simulink model "Lab6_dyskretny"  (R2017a)
settings: Solver=VariableStepAuto  StartTime=0.0  StopTime=10.0  FixedStep=0.01  RelTol=1e-3
values from neighbouring files (symbols this model uses):
  h = bodeplot(K)    [Lab1.m]    (also in Lab5.m = nyquistplot(K0); Lab6.m = h1)
libraries: cstblocks x2
settings Model: Creator=ishiguro  LastModifiedBy=ishiguro
settings DataIOCC: TimeSaveName=tout_dysk

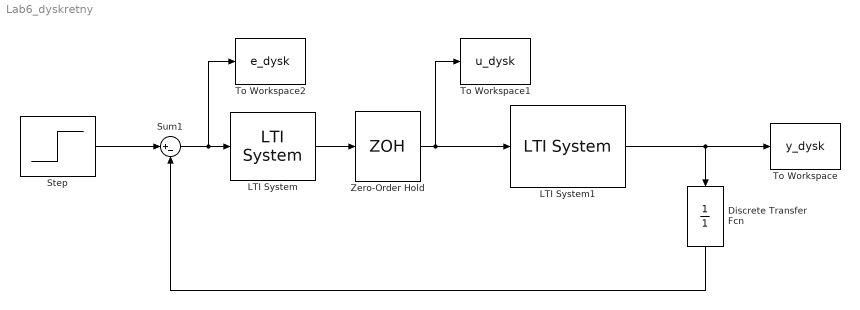
== system Lab6_dyskretny ==
  Discrete Transfer Fcn : DiscreteTransferFcn  Denominator=[1]  SampleTime=h
  LTI System : cstblocks/LTI System  sys=Kr  IC=[]
  LTI System1 : cstblocks/LTI System  sys=K  IC=[]
  Step : Step  Time=0  SampleTime=0
  Sum1 : Sum  Inputs=|+-
  To Workspace : ToWorkspace  VariableName=y_dysk  SampleTime=-1
  To Workspace1 : ToWorkspace  VariableName=u_dysk  SampleTime=-1
  To Workspace2 : ToWorkspace  VariableName=e_dysk  SampleTime=-1
  Zero-Order Hold : ZeroOrderHold  SampleTime=h
  wires:
  Sum1/1 -> To Workspace2/1, LTI System/1
  Step/1 -> Sum1/1
  LTI System1/1 -> Discrete Transfer Fcn/1, To Workspace/1
  Discrete Transfer Fcn/1 -> Sum1/2
  LTI System/1 -> Zero-Order Hold/1
  Zero-Order Hold/1 -> To Workspace1/1, LTI System1/1
